simulink model "Ejercicio1"  (R2025a)
settings: Solver=ode45  StartTime=0.0  StopTime=10.0  RelTol=1e-3
libraries: fuzblock x1
settings Model: Creator=zokra  LastModifiedBy=440G5

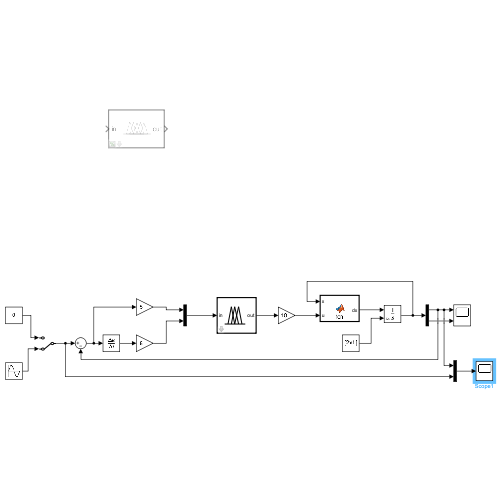
[thumbnail: Simulink's stored preview of the top-level diagram]
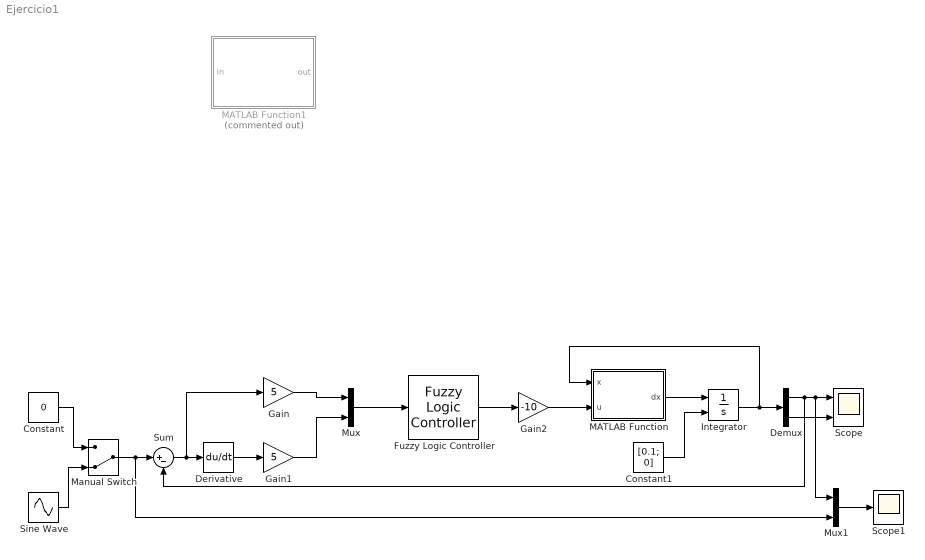
== system Ejercicio1 ==
  Constant : Constant  Value=0
  Constant1 : Constant  Value=[0.1; 0]
  Demux : Demux  Outputs=2
  Derivative : Derivative
  Fuzzy Logic Controller : fuzblock/Fuzzy Logic  Controller  FIS='25_rules_4.fis'  OutputSampleNumber=101  DataType=double  UseLookupTable=off  NumBreakpoints=10  FuzzifiedInputs=off  RuleFiringStrengths=off  RuleOutputs=off  AggregatedOutputs=off  SimulateUsing=Interpreted execution  OutOfRangeInputValueMessage=warning  NoRuleFiredMessage=warning  EmptyOutputFuzzySetMessage=warning
  Gain : Gain  Gain=5
  Gain1 : Gain  Gain=5
  Gain2 : Gain  Gain=-10
  Integrator : Integrator  InitialConditionSource=external
  MATLAB Function : MATLAB Function  TreatAsAtomicUnit=on
  MATLAB Function1 : MATLAB Function  Commented=on  TreatAsAtomicUnit=on  mask{DefuzzyMethod=COG, range_input_1=[-pi/2, pi/2], range_input_2=0, range_output=0}
      mask prompts: DefuzzyMethod "Defusificación"; range_input_1 "Rango Input 1"; range_input_2 "Rango Input 2"; range_output "Rango Output"
  Manual Switch : ManualSwitch  CurrentSetting=0
  Mux : Mux  Inputs=2
  Mux1 : Mux  Inputs=2
  Scope : Scope  NumInputPorts=2
      settings: ActiveDisplayYMinimum=-1.3075459669239078  ActiveDisplayYMaximum=1.2977307322664664
  Scope1 : Scope
      settings: ActiveDisplayYMinimum=-1.138168503669603  ActiveDisplayYMaximum=2.65744011714068
  Sine Wave : Sin  Amplitude=0.25  Frequency=4  SampleTime=0
  Sum : Sum  Inputs=|+-
  wires:
  Derivative/1 -> Gain1/1
  Gain/1 -> Mux/1
  Gain1/1 -> Mux/2
  Integrator/1 -> Demux/1, MATLAB Function/1(x)
  Constant1/1 -> Integrator/2
  Manual Switch/1 -> Mux1/2, Sum/1
  Sum/1 -> Gain/1, Derivative/1
  Mux1/1 -> Scope1/1
  Demux/1 -> Scope/1, Mux1/1, Sum/2
  Demux/2 -> Scope/2
  Sine Wave/1 -> Manual Switch/2
  Constant/1 -> Manual Switch/1
  MATLAB Function/1(dx) -> Integrator/1
  Gain2/1 -> MATLAB Function/2(u)
  Mux/1 -> Fuzzy Logic Controller/1
  Fuzzy Logic Controller/1 -> Gain2/1

== matlab function Ejercicio1/MATLAB Function ==
  data: x input; u input; dx output
function dx  = fcn(x, u)
g = 9.81;  
l = 1;     
m = 1;     
b = 0.5;   

x1 = x(1);  
x2 = x(2);

dx1 = x2;
dx2 = (g/l)*sin(x1) - (b/(m*l^2))*x2 + u/(m*l^2);

dx = [dx1; dx2];

y = x1;

== matlab function Ejercicio1/MATLAB Function1 ==
  data: in input; out output
function out = fcn(in)
range_input_1
out = in;
